simulink library "momentum_dump_lib"  (R2016b)
settings: Solver=VariableStepAuto  StartTime=0.0  StopTime=10.0  RelTol=1e-3
values from neighbouring files (symbols this model uses):
  fsw_params = init_fsw_params()    [momentum_unload_test_init.m]
settings Model: Creator=unsik  LastModifiedBy=evich

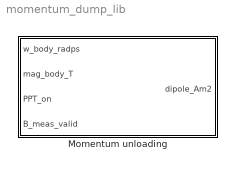
== system momentum_dump_lib ==
  Momentum unloading : Subsystem

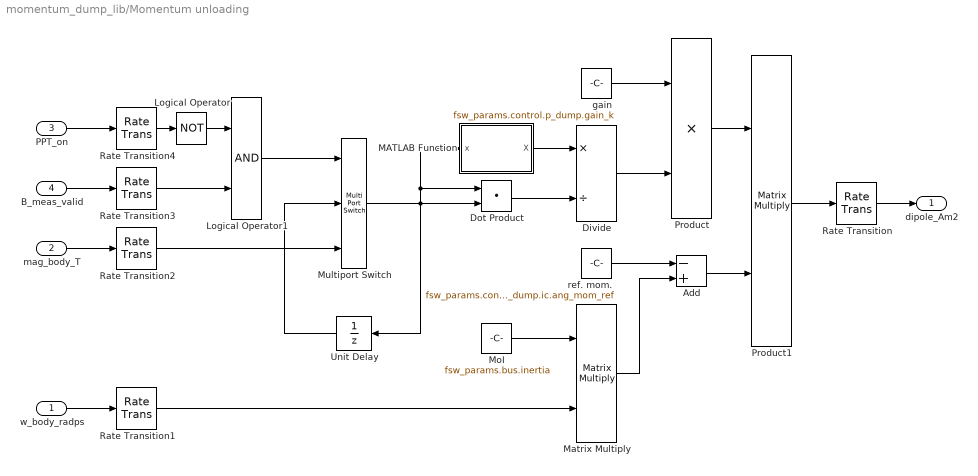
== system momentum_dump_lib/Momentum unloading ==
  w_body_radps : Inport
  mag_body_T : Inport  Port=2
  PPT_on : Inport  Port=3
  B_meas_valid : Inport  Port=4
  Add : Sum  Inputs=-+
  Divide : Product  Inputs=*/
  Dot Product : DotProduct  InputSameDT=on  OutDataTypeStr=Inherit: Inherit via internal rule
  Logical Operator : Logic  Operator=NOT  AllPortsSameDT=off  OutDataTypeStr=boolean
  Logical Operator1 : Logic  AllPortsSameDT=off  OutDataTypeStr=boolean
  MATLAB Function : MATLAB Function  TreatAsAtomicUnit=on
  Matrix Multiply : Product  Inputs=**  Multiplication=Matrix(*)
  MoI : Constant  Value=fsw_params.bus.inertia
  Multiport Switch : MultiPortSwitch  DataPortOrder=Zero-based contiguous  Inputs=2
  Product : Product  Inputs=**
  Product1 : Product  Inputs=**  Multiplication=Matrix(*)
  Rate Transition : RateTransition  X0=fsw_params.control.p_dump.ic.rt_dipole_Am2
  Rate Transition1 : RateTransition  X0=fsw_params.control.p_dump.ic.rt_w_body_radps  OutPortSampleTime=fsw_params.control.p_dump.sample_time_s
  Rate Transition2 : RateTransition  X0=fsw_params.control.p_dump.ic.rt_mag_body_T  OutPortSampleTime=fsw_params.control.p_dump.sample_time_s
  Rate Transition3 : RateTransition  X0=fsw_params.control.p_dump.ic.rt_B_meas_valid  OutPortSampleTime=fsw_params.control.p_dump.sample_time_s
  Rate Transition4 : RateTransition  X0=fsw_params.control.p_dump.ic.rt_PPT_on  OutPortSampleTime=fsw_params.control.p_dump.sample_time_s
  Unit Delay : UnitDelay  InitialCondition=fsw_params.control.p_dump.ic.delay  SampleTime=-1
  gain : Constant  Value=fsw_params.control.p_dump.gain_k
  ref. mom. : Constant  Value=fsw_params.control.p_dump.ic.ang_mom_ref
  dipole_Am2 : Outport
  wires:
  Logical Operator1/1 -> Multiport Switch/1
  Logical Operator/1 -> Logical Operator1/1
  Rate Transition3/1 -> Logical Operator1/2
  Rate Transition4/1 -> Logical Operator/1
  Rate Transition2/1 -> Multiport Switch/3
  Unit Delay/1 -> Multiport Switch/2
  PPT_on/1 -> Rate Transition4/1
  B_meas_valid/1 -> Rate Transition3/1
  mag_body_T/1 -> Rate Transition2/1
  Rate Transition/1 -> dipole_Am2/1
  Divide/1 -> Product/2
  Dot Product/1 -> Divide/2
  gain/1 -> Product/1
  Multiport Switch/1 -> Unit Delay/1, Dot Product/2, MATLAB Function/1(x), Dot Product/1
  w_body_radps/1 -> Rate Transition1/1
  Rate Transition1/1 -> Matrix Multiply/2
  ref. mom./1 -> Add/1
  Matrix Multiply/1 -> Add/2
  Product/1 -> Product1/1
  Add/1 -> Product1/2
  Product1/1 -> Rate Transition/1
  MATLAB Function/1(X) -> Divide/1
  MoI/1 -> Matrix Multiply/1

== matlab function momentum_dump_lib/Momentum unloading/MATLAB Function ==
  data: x input; X output
function X   = skew( x )
% UW HuskySat-1, ADCS Subsystem
% Last Update: E. Hansen 12.8.2017

%Transforms a vector into a skew symmetric matrix (Levi-Civita)
%--------------------------------------------------------------------------

X = [0 -x(3) x(2);x(3) 0 -x(1);-x(2) x(1) 0];
